simulink model "basic_pid"  (R2015a)
settings: Solver=ode45  StartTime=0.0  StopTime=10.0  RelTol=1e-3
model workspace (MAT data in the model file):
  J_L = 4.17e-06
  J_m = 0.015625
  K_a = 1.4
  K_d = 10
  K_i = 100
  K_p = 100
  K_t = 0.022879
  N = 1
  T_sample_control = 0.001
  b_L = 0.01
  b_m = 0.00045
  g = 9.8
  k_1 = 10
  k_2 = 0
  l = 0.25
  m = 0.25
  theta_c = 0
undefined symbols (not defined in the file): pid
libraries: simulink x4
settings Model: Creator=preston  LastModifiedBy=preston

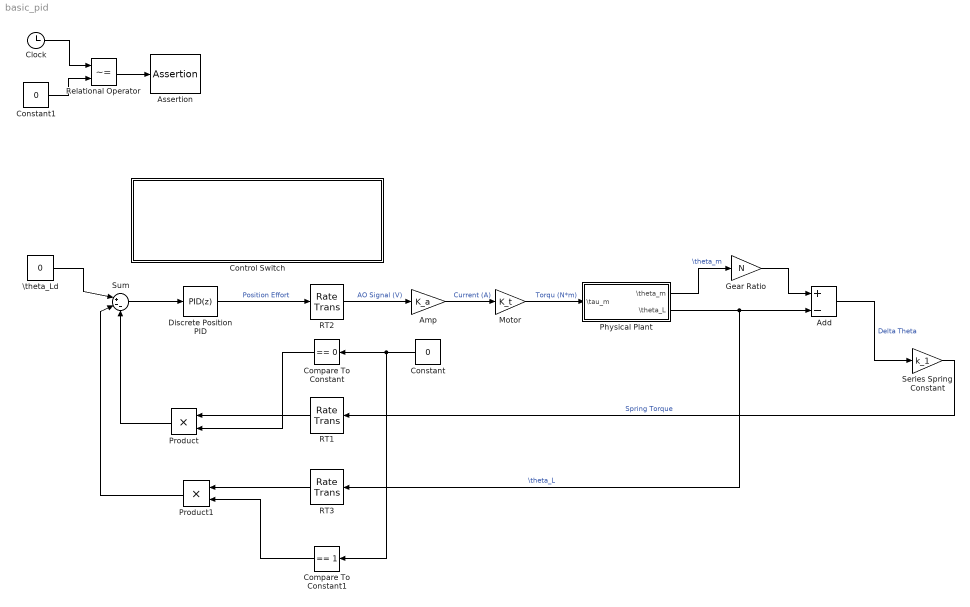
== system basic_pid ==
  Add : Sum  Inputs=+-
  Amp : Gain  Gain=K_a
  Assertion : Assertion  AssertionFailFcn=|  StopWhenAssertionFail=off
      | set_param(bdroot,'SimulationCommand','pause'),
      | disp(sprintf('\nSimulation paused.'))
  Clock : Clock
  Compare To Constant : simulink/Logic and Bit Operations/Compare To Constant  relop===  const=0  OutDataTypeStr=uint8
  Compare To Constant1 : simulink/Logic and Bit Operations/Compare To Constant  relop===  const=1  OutDataTypeStr=uint8
  Constant : Constant  Value=0
  Constant1 : Constant  Value=0
  Control Switch : Subsystem  DialogController=hmiCreateDDGDialog  IsWebBlock=on  mask(MathWorksWebBlock){webBlockId=a043e4fe-33d5-4f88-b2e3-ade745b31b59, webBlockType=discreteknob, ShowInLibBrowser=on, ShowInitialText=on, HMISrcModelName=basic_pid}
      mask prompts: webBlockId "WebBlock Id"; webBlockType "WebBlock Type"; HMISrcModelName "Source Model"
      mask Help: helpview([docroot '/mapfiles/simulink.map'], 'hmi_rotary_switch')
      mask Display:
      | model = bdroot(gcb);
      | if strcmp(get_param(model,'BlockDiagramType'), 'library')
      |     image([(matlabroot) '/toolbox/simulink/hmi/icons/DiscreteKnob.png']);
      | end
  Discrete Position PID : simulink/Continuous/PID Controller  Controller=PID  TimeDomain=Discrete-time  SampleTime=-1  IntegratorMethod=Backward Euler  FilterMethod=Forward Euler  Form=Parallel  UseFilter=off  ControllerParametersSource=internal  P=K_p  I=K_i  D=K_d  N=pid.N  InitialConditionSource=internal  InitialConditionForIntegrator=0  InitialConditionForFilter=0  ExternalReset=none  LimitOutput=off  UpperSaturationLimit=inf  LowerSaturationLimit=-inf  LinearizeAsGain=off  AntiWindupMode=none  Kb=1  TrackingMode=off  Kt=1  PParamMin=[]  PParamMax=[]  IParamMin=[]  IParamMax=[]  DParamMin=[]  DParamMax=[]  NParamMin=[]  NParamMax=[]  KbParamMin=[]  KbParamMax=[]  KtParamMin=[]  KtParamMax=[]  POutMin=[]  POutMax=[]  IOutMin=[]  IOutMax=[]  DOutMin=[]  DOutMax=[]  NOutMin=[]  NOutMax=[]  KbOutMin=[]  KbOutMax=[]  KtOutMin=[]  KtOutMax=[]  IntegratorOutMin=[]  IntegratorOutMax=[]  FilterOutMin=[]  FilterOutMax=[]  SumOutMin=[]  SumOutMax=[]  SumI1OutMin=[]  SumI1OutMax=[]  SumI2OutMin=[]  SumI2OutMax=[]  SumI3OutMin=[]  SumI3OutMax=[]  SumDOutMin=[]  SumDOutMax=[]  SaturationOutMin=[]  SaturationOutMax=[]  IntegratorContinuousStateAttributes=''  IntegratorStateMustResolveToSignalObject=off  IntegratorRTWStateStorageClass=Auto  FilterContinuousStateAttributes=''  FilterStateMustResolveToSignalObject=off  FilterRTWStateStorageClass=Auto  DifferentiatorICPrevScaledInput=0  DifferentiatorOutMin=[]  DifferentiatorOutMax=[]
  Gear Ratio : Gain  Gain=N
  Motor : Gain  Gain=K_t
  "Physical Plant " : Subsystem
  Product : Product
  Product1 : Product
  RT1 : RateTransition  OutPortSampleTime=T_sample_control
  RT2 : RateTransition
  RT3 : RateTransition  OutPortSampleTime=T_sample_control
  Relational Operator : RelationalOperator  Operator=~=  OutDataTypeStr=boolean
  Series Spring Constant : Gain  Gain=k_1
  Sum : Sum  Inputs=|+--
  \theta_Ld : Constant  Value=0
  wires:
  RT2/1 -> Amp/1  "AO Signal (V)"
  Discrete Position PID/1 -> RT2/1  "Position Effort"
  \theta_Ld/1 -> Sum/1
  RT1/1 -> Product/1
  Sum/1 -> Discrete Position PID/1
  Amp/1 -> Motor/1  "Current (A)"
  Motor/1 -> "Physical Plant "/1(\tau_m)  "Torqu (N*m)"
  Series Spring Constant/1 -> RT1/1  "Spring Torque"
  Add/1 -> Series Spring Constant/1  "Delta Theta"
  "Physical Plant "/1("\\theta_m ") -> Gear Ratio/1  "\\theta_m"
  Gear Ratio/1 -> Add/1
  "Physical Plant "/2(\theta_L) -> RT3/1, Add/2  "\\theta_L"
  RT3/1 -> Product1/1
  Product/1 -> Sum/3
  Product1/1 -> Sum/2
  Constant/1 -> Compare To Constant1/1, Compare To Constant/1
  Compare To Constant/1 -> Product/2
  Compare To Constant1/1 -> Product1/2
  Constant1/1 -> Relational Operator/2
  Clock/1 -> Relational Operator/1
  Relational Operator/1 -> Assertion/1

== system basic_pid/Control Switch ==

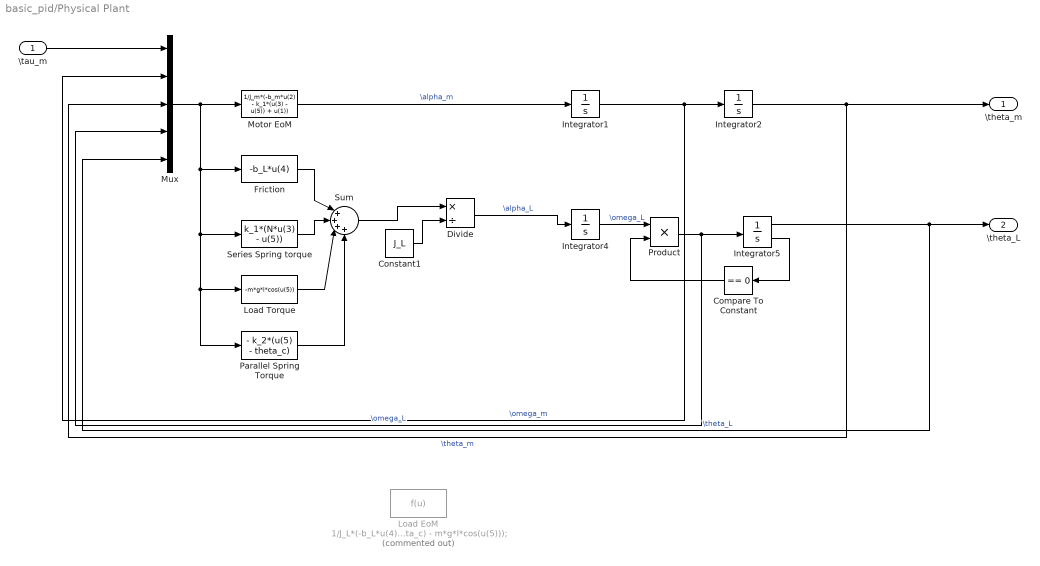
== system basic_pid/Physical Plant  ==
  \tau_m : Inport
  Compare To Constant : simulink/Logic and Bit Operations/Compare To Constant  relop===  const=0  OutDataTypeStr=boolean
  Constant1 : Constant  Value=J_L
  Divide : Product  Inputs=*/
  Friction : Fcn  Expr=-b_L*u(4)
  Integrator1 : Integrator
  Integrator2 : Integrator
  Integrator4 : Integrator
  Integrator5 : Integrator  LimitOutput=on  UpperSaturationLimit=pi/4  LowerSaturationLimit=-pi/4  ShowSaturationPort=on
  Load EoM : Fcn  Commented=on  Expr=1/J_L*(-b_L*u(4) + k_1*(u(3) - u(5)) - k_2*(u(5) - theta_c) - m*g*l*cos(u(5)));
  Load Torque : Fcn  Expr=-m*g*l*cos(u(5))
  Motor EoM : Fcn  Expr=1/J_m*(-b_m*u(2) - k_1*(u(3) - u(5)) + u(1))
  Mux : Mux  Inputs=5
  Parallel Spring Torque : Fcn  Expr=- k_2*(u(5) - theta_c)
  Product : Product
  Series Spring torque : Fcn  Expr=k_1*(N*u(3) - u(5))
  Sum : Sum  Inputs=|++++
  "\\theta_m " : Outport
  \theta_L : Outport  Port=2
  wires:
  Motor EoM/1 -> Integrator1/1  "\\alpha_m"
  Divide/1 -> Integrator4/1  "\\alpha_L"
  Integrator5/1 -> \theta_L/1, Mux/5  "\\theta_L"
  Mux/1 -> Series Spring torque/1, Parallel Spring Torque/1, Load Torque/1, Friction/1, Motor EoM/1
  \tau_m/1 -> Mux/1
  Constant1/1 -> Divide/2
  Sum/1 -> Divide/1
  Friction/1 -> Sum/1
  Series Spring torque/1 -> Sum/2
  Load Torque/1 -> Sum/3
  Integrator5/2 -> Compare To Constant/1
  Integrator4/1 -> Product/1  "\\omega_L"
  Compare To Constant/1 -> Product/2
  Product/1 -> Integrator5/1, Mux/4  "\\omega_L"
  Integrator1/1 -> Mux/2, Integrator2/1  "\\omega_m"
  Integrator2/1 -> Mux/3, "\\theta_m "/1  "\\theta_m"
  Parallel Spring Torque/1 -> Sum/4
